simulink library "lib_first_order_filter"  (R2023a)
settings: Solver=VariableStepAuto  StartTime=0.0  StopTime=10.0  RelTol=1e-3
libraries: lib_conversion x12, lib_resettable_unit_delay x2
settings Model: Creator=cav2ofo  LastModifiedBy=lenovo
settings OptimizationCC: ReuseModelBlockBuffer=off

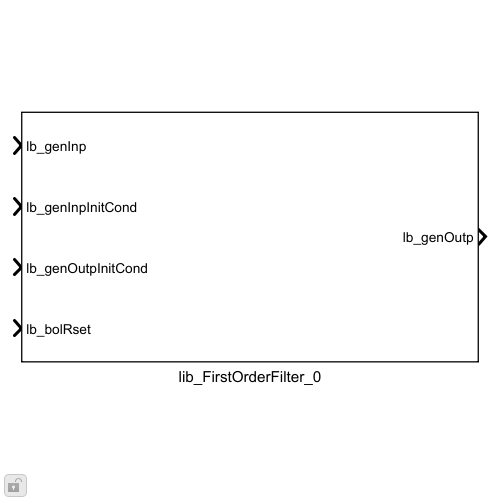
[thumbnail: Simulink's stored preview of the top-level diagram]
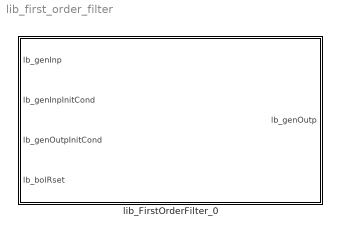
== system lib_first_order_filter ==
  lib_FirstOrderFilter_0 : Subsystem  mask{lb_parSampTime=0.01, lb_parTimeCnst=0.001, lb_parMaxTimeCnst=0, lb_parMinTimeCnst=0, lb_parMaxInpVal=1, lb_parInpVrntMaxVal=0, lb_parAccmDataType=fixdt(1,32,2^-25,0), lb_parIIntrDataTypeMode=Same of output, lb_parOutpDataType=fixdt(1,16,2^-3,0)}
      mask prompts: lb_parSampTime "Sampling time [s]:"; lb_parTimeCnst "Time constant [s]:"; lb_parMaxTimeCnst "Maximum time constant [s]:"; lb_parMinTimeCnst "Minimum time constant [s]:"; lb_parMaxInpVal "Maximum input value [iu]:"; lb_parInpVrntMaxVal "Maximum input variation [iu]:"; lb_parAccmDataType "Accumulator data type:"; lb_parIIntrDataTypeMode "Internal data types mode:"; lb_parOutpDataType "Output data type:"
      mask init:
      | slack = 1e-2; % slack variable
      | 
      | % Assign internal data types based on maximum values
      | lb_parCnst1 = (1+slack)*(double(lb_parTimeCnst)*2); % 2*Tc
      | if (double(lb_parTimeCnst)*2-double(lb_parSampTime)) >= 0 % 2Tc-Ts
      |     lb_parCnst2 = (1+slack)*(double(lb_parTimeCnst)*2-double(lb_parSampTime));
      | else
      |     lb_parCnst2 = (1-slack)*(double(lb_parTimeCnst)*2-double(lb_parSampTime));
      | end
      | lb_parCnst3 = (1+slack)*(double(lb_parTimeCnst)*2+double(lb_parSampTime));
      | if (double(lb_parTimeCnst)*2-double(lb_parSampTime)) >= 0 % (2Tc-Ts)/(2Tc+Ts)
      |     lb_parCnst4 = (1+slack)*((double(lb_parTimeCnst)*2-double(lb_parSampTime))/...
      |         (double(lb_parTimeCnst)*2+double(lb_parSampTime)));
      | else
      |     lb_parCnst4 = (1-slack)*((double(lb_parTimeCnst)*2-double(lb_parSampTime))/...
      |         (double(lb_parTimeCnst)*2+double(lb_parSampTime)));
      | end
      | lb_parCnst5 = (1+slack)*(double(lb_parSampTime)/...
      |     (double(lb_parTimeCnst)*2+double(lb_parSampTime))); % Ts/(2Tc+Ts)
      | 
      | % Assign data type for lib_Conversion_12
      | if lb_parMaxInpVal*2 <= (2^(16-1)-1)
      |     lb_parConv12DataType=Simulink.NumericType;
      |     lb_parConv12DataType.DataTypeMode= 'Fixed-point: unspecified scaling';
      |     lb_parConv12DataType.Signedness= 'Signed';
      |     lb_parConv12DataType.WordLength = 16;
      |     
      | else
      |     lb_parConv12DataType=Simulink.NumericType;
      |     lb_parConv12DataType.DataTypeMode= 'Fixed-point: unspecified scaling';
      |     lb_parConv12DataType.Signedness= 'Signed';
      |     lb_parConv12DataType.WordLength = 32;
      | end
      | lb_parConv12MaxVal = lb_parMaxInpVal*2;
      | 
      | %% Determine number of bits for internal data types
      | switch lb_parIIntrDataTypeMode
      |     case 'Same of output'
      |         temp.bitNum_scl = lb_parOutpDataType.WordLength;
      |     case '32-bit'
      |         temp.bitNum_scl = 32;
      | end
      | 
      | %% Compute data type for parameter cnst1=2*Tc
      | lb_parCnst1MaxVal = 2*lb_parMaxTimeCnst;
      | lb_parCnst1DataType = Simulink.NumericType;
      | lb_parCnst1DataType.DataTypeMode = 'Fixed-point: unspecified scaling';
      | lb_parCnst1DataType.Signedness = 'Unsigned';
      | lb_parCnst1DataType.WordLength = 16;
      | 
      | %% Compute data type for parameter cnst2=2*Tc+Ts
      | lb_parCnst2MaxVal = lb_parSampTime+2*lb_parMaxTimeCnst;
      | lb_parCnst2DataType = Simulink.NumericType;
      | lb_parCnst2DataType.DataTypeMode = 'Fixed-point: unspecified scaling';
      | lb_parCnst2DataType.Signedness = 'Unsigned';
      | lb_parCnst2DataType.WordLength = 16;
      | 
      | %% Compute data type for parameter cnst3=2*Tc-Ts
      | lb_parCnst3MaxVal = 2*lb_parMaxTimeCnst-lb_parSampTime;
      | lb_parCnst3DataType = Simulink.NumericType;
      | lb_parCnst3DataType.DataTypeMode = 'Fixed-point: unspecified scaling';
      | if lb_parCnst3MaxVal >= 0
      | lb_parCnst3DataType.Signedness = 'Unsigned';
      | else
      |    lb_parCnst3DataType.Signedness = 'Signed'; 
      | end
      | lb_parCnst3DataType.WordLength = 16;
      | 
      | %% Compute data type for parameter cnst4=Ts/(2*Tc+Ts)
      | lb_parCnst4MaxVal = lb_parSampTime/(2*lb_parMinTimeCnst+lb_parSampTime);
      | lb_parCnst4DataType = Simulink.NumericType;
      | lb_parCnst4DataType.DataTypeMode = 'Fixed-point: unspecified scaling';
      | lb_parCnst4DataType.Signedness = 'Unsigned';
      | lb_parCnst4DataType.WordLength = 16;
      | 
      | %% Compute data type for parameter cnst5=(2*Tc-Ts)/(2Tc+Ts)
      | temp.TimeCnst_vec = linspace(lb_parMinTimeCnst,lb_parMaxTimeCnst,10000);
      | lb_parCnst5MaxVal = max((2*temp.TimeCnst_vec-lb_parSampTime)./...
      |     (2*temp.TimeCnst_vec+lb_parSampTime))*1.1;
      | lb_parCnst5DataType = Simulink.NumericType;
      | lb_parCnst5DataType.DataTypeMode = 'Fixed-point: unspecified scaling';
      | if lb_parCnst5MaxVal >= 0
      | lb_parCnst5DataType.Signedness = 'Unsigned';
      | else
      |    lb_parCnst5DataType.Signedness = 'Signed'; 
      | end
      | lb_parCnst5DataType.WordLength = 16;
      | 
      | %% Compute data type for input variation
      | lb_parInpVrntDataType = Simulink.NumericType;
      | lb_parInpVrntDataType.DataTypeMode = 'Fixed-point: unspecified scaling';
      | lb_parInpVrntDataType.Signedness = 'Signed';
      | lb_parInpVrntDataType.WordLength = temp.bitNum_scl;
      | 
      | %% Compute data type for feedfoward term of output
      | lb_parFdfwTermMaxVal = lb_parInpVrntMaxVal*lb_parCnst5MaxVal;
      | lb_parFdfwTermDataType = Simulink.NumericType;
      | lb_parFdfwTermDataType.DataTypeMode = 'Fixed-point: unspecified scaling';
      | lb_parFdfwTermDataType.Signedness = 'Signed';
      | lb_parFdfwTermDataType.WordLength = temp.bitNum_scl;
      | 
      | %% Compute data type for feedback term of output
      | lb_parFdbkTermMaxVal = lb_parMaxInpVal*lb_parCnst5MaxVal;
      | lb_parFdbkTermDataType = Simulink.NumericType;
      | lb_parFdbkTermDataType.DataTypeMode = 'Fixed-point: unspecified scaling';
      | lb_parFdbkTermDataType.Signedness = lb_parOutpDataType.Signedness;
      | lb_parFdbkTermDataType.WordLength = temp.bitNum_scl;
      | 
      | %% Compute data type for feedbacked output
      | lb_parAccmDataTypeMaxVal =  lb_parFdfwTermMaxVal+lb_parFdbkTermMaxVal;
      | lb_parAccmDataType = Simulink.NumericType;
      | lb_parAccmDataType.DataTypeMode = 'Fixed-point: unspecified scaling';
      | lb_parAccmDataType.Signedness = 'Signed';
      | lb_parAccmDataType.WordLength = temp.bitNum_scl;
      | 
      | clear temp;
      mask TypeOptions lb_parIIntrDataTypeMode: Same of output | 32-bit
      mask DialogControl DescGroupVar Prompt: VHIT control library
      mask DialogControl DescTextVar Prompt: First order filter
      mask DialogControl Container3 Prompt: Data type

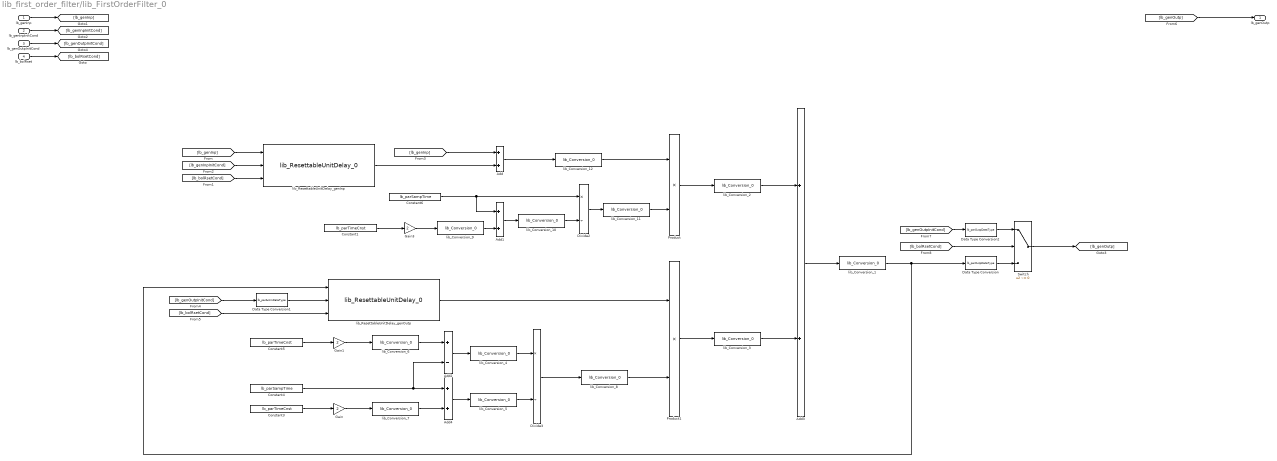
== system lib_first_order_filter/lib_FirstOrderFilter_0 ==
  lb_genInp : Inport
  lb_genInpInitCond : Inport  Port=2
  lb_genOutpInitCond : Inport  Port=3
  lb_bolRset : Inport  Port=4
  Add{,1,3..4} (4 alike) : Sum  OutDataTypeStr=Inherit: Inherit via back propagation
  Add2 : Sum  Inputs=+-  OutDataTypeStr=Inherit: Inherit via back propagation
  Constant1 : Constant  Value=lb_parTimeCnst
  Constant3 : Constant  Value=lb_parTimeCnst
  Constant4 : Constant  Value=lb_parSampTime
  Constant5 : Constant  Value=lb_parTimeCnst
  Constant6 : Constant  Value=lb_parSampTime
  Data Type Conversion : DataTypeConversion  OutDataTypeStr=lb_parOutpDataType  SaturateOnIntegerOverflow=off  RndMeth=Floor
  Data Type Conversion1 : DataTypeConversion  OutDataTypeStr=lb_parAccmDataType  SaturateOnIntegerOverflow=off  RndMeth=Floor
  Data Type Conversion2 : DataTypeConversion  OutDataTypeStr=lb_parOutpDataType  SaturateOnIntegerOverflow=off  RndMeth=Floor
  Divide2 : Product  Inputs=*/  OutDataTypeStr=Inherit: Inherit via back propagation
  Divide3 : Product  Inputs=*/  OutDataTypeStr=Inherit: Inherit via back propagation
  Gain : Gain  Gain=2  OutDataTypeStr=Inherit: Inherit via back propagation
  Gain1 : Gain  Gain=2  OutDataTypeStr=Inherit: Inherit via back propagation
  Gain3 : Gain  Gain=2  OutDataTypeStr=Inherit: Inherit via back propagation
  Product : Product  OutDataTypeStr=Inherit: Inherit via back propagation
  Product1 : Product  OutDataTypeStr=Inherit: Inherit via back propagation
  Switch : Switch  Criteria=u2 ~= 0  SaturateOnIntegerOverflow=off  InputSameDT=off
  lib_Conversion_1 : lib_conversion/lib_Conversion_0  lb_parDataType=lb_parAccmDataType  lb_parOutpMaxVal=[]  lb_parOutpMinVal=[]  lb_parSatFlag=off
  lib_Conversion_10 : lib_conversion/lib_Conversion_0  lb_parDataType=fixdt(1,16)  lb_parOutpMaxVal=lb_parCnst3  lb_parOutpMinVal=[]  lb_parSatFlag=off
  lib_Conversion_11 : lib_conversion/lib_Conversion_0  lb_parDataType=fixdt(1,16)  lb_parOutpMaxVal=lb_parCnst5  lb_parOutpMinVal=[]  lb_parSatFlag=off
  lib_Conversion_12 : lib_conversion/lib_Conversion_0  lb_parDataType=lb_parConv12DataType  lb_parOutpMaxVal=lb_parConv12MaxVal  lb_parOutpMinVal=[]  lb_parSatFlag=off
  lib_Conversion_2 : lib_conversion/lib_Conversion_0  lb_parDataType=lb_parAccmDataType  lb_parOutpMaxVal=[]  lb_parOutpMinVal=[]  lb_parSatFlag=off
  lib_Conversion_3 : lib_conversion/lib_Conversion_0  lb_parDataType=lb_parOutpDataType  lb_parOutpMaxVal=[]  lb_parOutpMinVal=[]  lb_parSatFlag=off
  lib_Conversion_4 : lib_conversion/lib_Conversion_0  lb_parDataType=fixdt(1,16)  lb_parOutpMaxVal=lb_parCnst2  lb_parOutpMinVal=[]  lb_parSatFlag=off
  lib_Conversion_5 : lib_conversion/lib_Conversion_0  lb_parDataType=fixdt(1,16)  lb_parOutpMaxVal=lb_parCnst3  lb_parOutpMinVal=[]  lb_parSatFlag=off
  lib_Conversion_6 : lib_conversion/lib_Conversion_0  lb_parDataType=fixdt(1,16)  lb_parOutpMaxVal=lb_parCnst1  lb_parOutpMinVal=[]  lb_parSatFlag=off
  lib_Conversion_7 : lib_conversion/lib_Conversion_0  lb_parDataType=fixdt(1,16)  lb_parOutpMaxVal=lb_parCnst1  lb_parOutpMinVal=[]  lb_parSatFlag=off
  lib_Conversion_8 : lib_conversion/lib_Conversion_0  lb_parDataType=fixdt(1,16)  lb_parOutpMaxVal=lb_parCnst4  lb_parOutpMinVal=[]  lb_parSatFlag=off
  lib_Conversion_9 : lib_conversion/lib_Conversion_0  lb_parDataType=fixdt(1,16)  lb_parOutpMaxVal=lb_parCnst1  lb_parOutpMinVal=[]  lb_parSatFlag=off
  lib_ResettableUnitDelay_genInp : lib_resettable_unit_delay/lib_ResettableUnitDelay_0
      settings: LibrarySourceBlock=vhit_control_library/lib_ResettableUnitDelay_0
  lib_ResettableUnitDelay_genOutp : lib_resettable_unit_delay/lib_ResettableUnitDelay_0
      settings: LibrarySourceBlock=vhit_control_library/lib_ResettableUnitDelay_0
  lb_genOutp : Outport
  wires:
  lib_Conversion_3/1 -> Add3/2
  lib_Conversion_2/1 -> Add3/1
  lb_bolRset/1 -> [lb_bolRsetCond]
  lb_genInpInitCond/1 -> [lb_genInpInitCond]
  lb_genInp/1 -> [lb_genInp]
  [lb_bolRsetCond] -> lib_ResettableUnitDelay_genInp/3
  [lb_genInpInitCond] -> lib_ResettableUnitDelay_genInp/2
  [lb_genInp] -> lib_ResettableUnitDelay_genInp/1
  lb_genOutpInitCond/1 -> [lb_genOutpInitCond]
  Add/1 -> lib_Conversion_12/1
  lib_ResettableUnitDelay_genInp/1 -> Add/2
  [lb_genInp] -> Add/1
  Product/1 -> lib_Conversion_2/1
  Product1/1 -> lib_Conversion_3/1
  lib_ResettableUnitDelay_genOutp/1 -> Product1/1
  [lb_genOutpInitCond] -> Data Type Conversion1/1
  [lb_bolRsetCond] -> lib_ResettableUnitDelay_genOutp/3
  Add3/1 -> lib_Conversion_1/1
  [lb_genOutp] -> lb_genOutp/1
  lib_Conversion_1/1 -> lib_ResettableUnitDelay_genOutp/1, Data Type Conversion/1
  Constant1/1 -> Gain3/1
  Constant6/1 -> Add1/1, Divide2/1
  Divide2/1 -> lib_Conversion_11/1
  Add1/1 -> lib_Conversion_10/1
  lib_Conversion_10/1 -> Divide2/2
  Gain3/1 -> lib_Conversion_9/1
  lib_Conversion_11/1 -> Product/2
  Divide3/1 -> lib_Conversion_8/1
  Add2/1 -> lib_Conversion_4/1
  Constant3/1 -> Gain/1
  Gain/1 -> lib_Conversion_7/1
  lib_Conversion_4/1 -> Divide3/1
  Constant4/1 -> Add4/1, Add2/2
  Constant5/1 -> Gain1/1
  Gain1/1 -> lib_Conversion_6/1
  lib_Conversion_5/1 -> Divide3/2
  Add4/1 -> lib_Conversion_5/1
  lib_Conversion_8/1 -> Product1/2
  lib_Conversion_6/1 -> Add2/1
  lib_Conversion_7/1 -> Add4/2
  lib_Conversion_9/1 -> Add1/2
  Data Type Conversion1/1 -> lib_ResettableUnitDelay_genOutp/2
  lib_Conversion_12/1 -> Product/1
  Data Type Conversion/1 -> Switch/3
  [lb_genOutpInitCond] -> Data Type Conversion2/1
  Data Type Conversion2/1 -> Switch/1
  Switch/1 -> [lb_genOutp]
  [lb_bolRsetCond] -> Switch/2
